simulink model "RunningLEDExample"  (R2015a)
settings: Solver=ode3  SolverMode=SingleTasking  StartTime=0.0  StopTime=inf  FixedStep=Ts  RelTol=1e-3
undefined symbols (not defined in the file): Ts
libraries: simulink x1
(part 2 of 2)

== system RunningLEDExample/Subsystem7/Subsystem3 ==
  In1 : Inport
  Constant4 : Constant  Value=15  OutDataTypeStr=uint8
  Constant5 : Constant  Value=0  OutDataTypeStr=uint8
  If : If  IfExpression=u1 == 81
  If Action Subsystem : Subsystem  TreatAsAtomicUnit=on
  If Action Subsystem1 : Subsystem  TreatAsAtomicUnit=on
  Merge : Merge
  Out1 : Outport  OutDataTypeStr=uint8
  wires:
  If/1 -> If Action Subsystem/Action
  If/2 -> If Action Subsystem1/Action
  In1/1 -> If/1
  Constant5/1 -> If Action Subsystem1/1(In1)
  Merge/1 -> Out1/1
  Constant4/1 -> If Action Subsystem/1(In1)
  If Action Subsystem/1(Out1) -> Merge/1
  If Action Subsystem1/1(Out1) -> Merge/2

== system RunningLEDExample/Subsystem7/Subsystem4 ==
  In1 : Inport
  Constant4 : Constant  Value=15  OutDataTypeStr=uint8
  Constant5 : Constant  Value=0  OutDataTypeStr=uint8
  If : If  IfExpression=u1 == 82
  If Action Subsystem : Subsystem  TreatAsAtomicUnit=on
  If Action Subsystem1 : Subsystem  TreatAsAtomicUnit=on
  Merge : Merge
  Out1 : Outport  OutDataTypeStr=uint8
  wires:
  If/1 -> If Action Subsystem/Action
  If/2 -> If Action Subsystem1/Action
  In1/1 -> If/1
  Constant5/1 -> If Action Subsystem1/1(In1)
  Merge/1 -> Out1/1
  Constant4/1 -> If Action Subsystem/1(In1)
  If Action Subsystem/1(Out1) -> Merge/1
  If Action Subsystem1/1(Out1) -> Merge/2

== system RunningLEDExample/Subsystem8/Subsystem ==
  In1 : Inport
  Constant4 : Constant  Value=15  OutDataTypeStr=uint8
  Constant5 : Constant  Value=0  OutDataTypeStr=uint8
  If : If  IfExpression=u1 == 96
  If Action Subsystem : Subsystem  TreatAsAtomicUnit=on
  If Action Subsystem1 : Subsystem  TreatAsAtomicUnit=on
  Merge : Merge
  Out1 : Outport  OutDataTypeStr=uint8
  wires:
  If/1 -> If Action Subsystem/Action
  If/2 -> If Action Subsystem1/Action
  In1/1 -> If/1
  Constant5/1 -> If Action Subsystem1/1(In1)
  Merge/1 -> Out1/1
  Constant4/1 -> If Action Subsystem/1(In1)
  If Action Subsystem/1(Out1) -> Merge/1
  If Action Subsystem1/1(Out1) -> Merge/2

== system RunningLEDExample/Subsystem8/Subsystem3 ==
  In1 : Inport
  Constant4 : Constant  Value=15  OutDataTypeStr=uint8
  Constant5 : Constant  Value=0  OutDataTypeStr=uint8
  If : If  IfExpression=u1 == 97
  If Action Subsystem : Subsystem  TreatAsAtomicUnit=on
  If Action Subsystem1 : Subsystem  TreatAsAtomicUnit=on
  Merge : Merge
  Out1 : Outport  OutDataTypeStr=uint8
  wires:
  If/1 -> If Action Subsystem/Action
  If/2 -> If Action Subsystem1/Action
  In1/1 -> If/1
  Constant5/1 -> If Action Subsystem1/1(In1)
  Merge/1 -> Out1/1
  Constant4/1 -> If Action Subsystem/1(In1)
  If Action Subsystem/1(Out1) -> Merge/1
  If Action Subsystem1/1(Out1) -> Merge/2

== system RunningLEDExample/Subsystem8/Subsystem4 ==
  In1 : Inport
  Constant4 : Constant  Value=15  OutDataTypeStr=uint8
  Constant5 : Constant  Value=0  OutDataTypeStr=uint8
  If : If  IfExpression=u1 == 98
  If Action Subsystem : Subsystem  TreatAsAtomicUnit=on
  If Action Subsystem1 : Subsystem  TreatAsAtomicUnit=on
  Merge : Merge
  Out1 : Outport  OutDataTypeStr=uint8
  wires:
  If/1 -> If Action Subsystem/Action
  If/2 -> If Action Subsystem1/Action
  In1/1 -> If/1
  Constant5/1 -> If Action Subsystem1/1(In1)
  Merge/1 -> Out1/1
  Constant4/1 -> If Action Subsystem/1(In1)
  If Action Subsystem/1(Out1) -> Merge/1
  If Action Subsystem1/1(Out1) -> Merge/2

== system RunningLEDExample/Subsystem9/Subsystem ==
  In1 : Inport
  Constant4 : Constant  Value=15  OutDataTypeStr=uint8
  Constant5 : Constant  Value=0  OutDataTypeStr=uint8
  If : If  IfExpression=u1 == 112
  If Action Subsystem : Subsystem  TreatAsAtomicUnit=on
  If Action Subsystem1 : Subsystem  TreatAsAtomicUnit=on
  Merge : Merge
  Out1 : Outport  OutDataTypeStr=uint8
  wires:
  If/1 -> If Action Subsystem/Action
  If/2 -> If Action Subsystem1/Action
  In1/1 -> If/1
  Constant5/1 -> If Action Subsystem1/1(In1)
  Merge/1 -> Out1/1
  Constant4/1 -> If Action Subsystem/1(In1)
  If Action Subsystem/1(Out1) -> Merge/1
  If Action Subsystem1/1(Out1) -> Merge/2

== system RunningLEDExample/Subsystem9/Subsystem3 ==
  In1 : Inport
  Constant4 : Constant  Value=15  OutDataTypeStr=uint8
  Constant5 : Constant  Value=0  OutDataTypeStr=uint8
  If : If  IfExpression=u1 == 113
  If Action Subsystem : Subsystem  TreatAsAtomicUnit=on
  If Action Subsystem1 : Subsystem  TreatAsAtomicUnit=on
  Merge : Merge
  Out1 : Outport  OutDataTypeStr=uint8
  wires:
  If/1 -> If Action Subsystem/Action
  If/2 -> If Action Subsystem1/Action
  In1/1 -> If/1
  Constant5/1 -> If Action Subsystem1/1(In1)
  Merge/1 -> Out1/1
  Constant4/1 -> If Action Subsystem/1(In1)
  If Action Subsystem/1(Out1) -> Merge/1
  If Action Subsystem1/1(Out1) -> Merge/2

== system RunningLEDExample/Subsystem9/Subsystem4 ==
  In1 : Inport
  Constant4 : Constant  Value=15  OutDataTypeStr=uint8
  Constant5 : Constant  Value=0  OutDataTypeStr=uint8
  If : If  IfExpression=u1 == 114
  If Action Subsystem : Subsystem  TreatAsAtomicUnit=on
  If Action Subsystem1 : Subsystem  TreatAsAtomicUnit=on
  Merge : Merge
  Out1 : Outport  OutDataTypeStr=uint8
  wires:
  If/1 -> If Action Subsystem/Action
  If/2 -> If Action Subsystem1/Action
  In1/1 -> If/1
  Constant5/1 -> If Action Subsystem1/1(In1)
  Merge/1 -> Out1/1
  Constant4/1 -> If Action Subsystem/1(In1)
  If Action Subsystem/1(Out1) -> Merge/1
  If Action Subsystem1/1(Out1) -> Merge/2

== system RunningLEDExample/Subsystem1/Subsystem/If Action Subsystem ==
  In1 : Inport
  Action Port : ActionPort  ActionType=then
  Out1 : Outport  OutDataTypeStr=uint8
  wires:
  In1/1 -> Out1/1

== system RunningLEDExample/Subsystem1/Subsystem/If Action Subsystem1 ==
  In1 : Inport
  Action Port : ActionPort  ActionType=else
  Out1 : Outport  OutDataTypeStr=uint8
  wires:
  In1/1 -> Out1/1

== system RunningLEDExample/Subsystem1/Subsystem3/If Action Subsystem ==
  In1 : Inport
  Action Port : ActionPort  ActionType=then
  Out1 : Outport  OutDataTypeStr=uint8
  wires:
  In1/1 -> Out1/1

== system RunningLEDExample/Subsystem1/Subsystem3/If Action Subsystem1 ==
  In1 : Inport
  Action Port : ActionPort  ActionType=else
  Out1 : Outport  OutDataTypeStr=uint8
  wires:
  In1/1 -> Out1/1

== system RunningLEDExample/Subsystem1/Subsystem4/If Action Subsystem ==
  In1 : Inport
  Action Port : ActionPort  ActionType=then
  Out1 : Outport  OutDataTypeStr=uint8
  wires:
  In1/1 -> Out1/1

== system RunningLEDExample/Subsystem1/Subsystem4/If Action Subsystem1 ==
  In1 : Inport
  Action Port : ActionPort  ActionType=else
  Out1 : Outport  OutDataTypeStr=uint8
  wires:
  In1/1 -> Out1/1

== system RunningLEDExample/Subsystem10/Subsystem/If Action Subsystem ==
  In1 : Inport
  Action Port : ActionPort  ActionType=then
  Out1 : Outport  OutDataTypeStr=uint8
  wires:
  In1/1 -> Out1/1

== system RunningLEDExample/Subsystem10/Subsystem/If Action Subsystem1 ==
  In1 : Inport
  Action Port : ActionPort  ActionType=else
  Out1 : Outport  OutDataTypeStr=uint8
  wires:
  In1/1 -> Out1/1

== system RunningLEDExample/Subsystem10/Subsystem3/If Action Subsystem ==
  In1 : Inport
  Action Port : ActionPort  ActionType=then
  Out1 : Outport  OutDataTypeStr=uint8
  wires:
  In1/1 -> Out1/1

== system RunningLEDExample/Subsystem10/Subsystem3/If Action Subsystem1 ==
  In1 : Inport
  Action Port : ActionPort  ActionType=else
  Out1 : Outport  OutDataTypeStr=uint8
  wires:
  In1/1 -> Out1/1

== system RunningLEDExample/Subsystem10/Subsystem4/If Action Subsystem ==
  In1 : Inport
  Action Port : ActionPort  ActionType=then
  Out1 : Outport  OutDataTypeStr=uint8
  wires:
  In1/1 -> Out1/1

== system RunningLEDExample/Subsystem10/Subsystem4/If Action Subsystem1 ==
  In1 : Inport
  Action Port : ActionPort  ActionType=else
  Out1 : Outport  OutDataTypeStr=uint8
  wires:
  In1/1 -> Out1/1

== system RunningLEDExample/Subsystem11/Subsystem/If Action Subsystem ==
  In1 : Inport
  Action Port : ActionPort  ActionType=then
  Out1 : Outport  OutDataTypeStr=uint8
  wires:
  In1/1 -> Out1/1

== system RunningLEDExample/Subsystem11/Subsystem/If Action Subsystem1 ==
  In1 : Inport
  Action Port : ActionPort  ActionType=else
  Out1 : Outport  OutDataTypeStr=uint8
  wires:
  In1/1 -> Out1/1

== system RunningLEDExample/Subsystem11/Subsystem3/If Action Subsystem ==
  In1 : Inport
  Action Port : ActionPort  ActionType=then
  Out1 : Outport  OutDataTypeStr=uint8
  wires:
  In1/1 -> Out1/1

== system RunningLEDExample/Subsystem11/Subsystem3/If Action Subsystem1 ==
  In1 : Inport
  Action Port : ActionPort  ActionType=else
  Out1 : Outport  OutDataTypeStr=uint8
  wires:
  In1/1 -> Out1/1

== system RunningLEDExample/Subsystem11/Subsystem4/If Action Subsystem ==
  In1 : Inport
  Action Port : ActionPort  ActionType=then
  Out1 : Outport  OutDataTypeStr=uint8
  wires:
  In1/1 -> Out1/1

== system RunningLEDExample/Subsystem11/Subsystem4/If Action Subsystem1 ==
  In1 : Inport
  Action Port : ActionPort  ActionType=else
  Out1 : Outport  OutDataTypeStr=uint8
  wires:
  In1/1 -> Out1/1

== system RunningLEDExample/Subsystem12/Subsystem/If Action Subsystem ==
  In1 : Inport
  Action Port : ActionPort  ActionType=then
  Out1 : Outport  OutDataTypeStr=uint8
  wires:
  In1/1 -> Out1/1

== system RunningLEDExample/Subsystem12/Subsystem/If Action Subsystem1 ==
  In1 : Inport
  Action Port : ActionPort  ActionType=else
  Out1 : Outport  OutDataTypeStr=uint8
  wires:
  In1/1 -> Out1/1

== system RunningLEDExample/Subsystem12/Subsystem3/If Action Subsystem ==
  In1 : Inport
  Action Port : ActionPort  ActionType=then
  Out1 : Outport  OutDataTypeStr=uint8
  wires:
  In1/1 -> Out1/1

== system RunningLEDExample/Subsystem12/Subsystem3/If Action Subsystem1 ==
  In1 : Inport
  Action Port : ActionPort  ActionType=else
  Out1 : Outport  OutDataTypeStr=uint8
  wires:
  In1/1 -> Out1/1

== system RunningLEDExample/Subsystem12/Subsystem4/If Action Subsystem ==
  In1 : Inport
  Action Port : ActionPort  ActionType=then
  Out1 : Outport  OutDataTypeStr=uint8
  wires:
  In1/1 -> Out1/1

== system RunningLEDExample/Subsystem12/Subsystem4/If Action Subsystem1 ==
  In1 : Inport
  Action Port : ActionPort  ActionType=else
  Out1 : Outport  OutDataTypeStr=uint8
  wires:
  In1/1 -> Out1/1

== system RunningLEDExample/Subsystem13/Subsystem/If Action Subsystem ==
  In1 : Inport
  Action Port : ActionPort  ActionType=then
  Out1 : Outport  OutDataTypeStr=uint8
  wires:
  In1/1 -> Out1/1

== system RunningLEDExample/Subsystem13/Subsystem/If Action Subsystem1 ==
  In1 : Inport
  Action Port : ActionPort  ActionType=else
  Out1 : Outport  OutDataTypeStr=uint8
  wires:
  In1/1 -> Out1/1

== system RunningLEDExample/Subsystem13/Subsystem3/If Action Subsystem ==
  In1 : Inport
  Action Port : ActionPort  ActionType=then
  Out1 : Outport  OutDataTypeStr=uint8
  wires:
  In1/1 -> Out1/1

== system RunningLEDExample/Subsystem13/Subsystem3/If Action Subsystem1 ==
  In1 : Inport
  Action Port : ActionPort  ActionType=else
  Out1 : Outport  OutDataTypeStr=uint8
  wires:
  In1/1 -> Out1/1

== system RunningLEDExample/Subsystem13/Subsystem4/If Action Subsystem ==
  In1 : Inport
  Action Port : ActionPort  ActionType=then
  Out1 : Outport  OutDataTypeStr=uint8
  wires:
  In1/1 -> Out1/1

== system RunningLEDExample/Subsystem13/Subsystem4/If Action Subsystem1 ==
  In1 : Inport
  Action Port : ActionPort  ActionType=else
  Out1 : Outport  OutDataTypeStr=uint8
  wires:
  In1/1 -> Out1/1

== system RunningLEDExample/Subsystem14/Subsystem/If Action Subsystem ==
  In1 : Inport
  Action Port : ActionPort  ActionType=then
  Out1 : Outport  OutDataTypeStr=uint8
  wires:
  In1/1 -> Out1/1

== system RunningLEDExample/Subsystem14/Subsystem/If Action Subsystem1 ==
  In1 : Inport
  Action Port : ActionPort  ActionType=else
  Out1 : Outport  OutDataTypeStr=uint8
  wires:
  In1/1 -> Out1/1

== system RunningLEDExample/Subsystem14/Subsystem3/If Action Subsystem ==
  In1 : Inport
  Action Port : ActionPort  ActionType=then
  Out1 : Outport  OutDataTypeStr=uint8
  wires:
  In1/1 -> Out1/1

== system RunningLEDExample/Subsystem14/Subsystem3/If Action Subsystem1 ==
  In1 : Inport
  Action Port : ActionPort  ActionType=else
  Out1 : Outport  OutDataTypeStr=uint8
  wires:
  In1/1 -> Out1/1

== system RunningLEDExample/Subsystem14/Subsystem4/If Action Subsystem ==
  In1 : Inport
  Action Port : ActionPort  ActionType=then
  Out1 : Outport  OutDataTypeStr=uint8
  wires:
  In1/1 -> Out1/1

== system RunningLEDExample/Subsystem14/Subsystem4/If Action Subsystem1 ==
  In1 : Inport
  Action Port : ActionPort  ActionType=else
  Out1 : Outport  OutDataTypeStr=uint8
  wires:
  In1/1 -> Out1/1

== system RunningLEDExample/Subsystem15/Subsystem/If Action Subsystem ==
  In1 : Inport
  Action Port : ActionPort  ActionType=then
  Out1 : Outport  OutDataTypeStr=uint8
  wires:
  In1/1 -> Out1/1

== system RunningLEDExample/Subsystem15/Subsystem/If Action Subsystem1 ==
  In1 : Inport
  Action Port : ActionPort  ActionType=else
  Out1 : Outport  OutDataTypeStr=uint8
  wires:
  In1/1 -> Out1/1

== system RunningLEDExample/Subsystem15/Subsystem3/If Action Subsystem ==
  In1 : Inport
  Action Port : ActionPort  ActionType=then
  Out1 : Outport  OutDataTypeStr=uint8
  wires:
  In1/1 -> Out1/1

== system RunningLEDExample/Subsystem15/Subsystem3/If Action Subsystem1 ==
  In1 : Inport
  Action Port : ActionPort  ActionType=else
  Out1 : Outport  OutDataTypeStr=uint8
  wires:
  In1/1 -> Out1/1

== system RunningLEDExample/Subsystem15/Subsystem4/If Action Subsystem ==
  In1 : Inport
  Action Port : ActionPort  ActionType=then
  Out1 : Outport  OutDataTypeStr=uint8
  wires:
  In1/1 -> Out1/1

== system RunningLEDExample/Subsystem15/Subsystem4/If Action Subsystem1 ==
  In1 : Inport
  Action Port : ActionPort  ActionType=else
  Out1 : Outport  OutDataTypeStr=uint8
  wires:
  In1/1 -> Out1/1

== system RunningLEDExample/Subsystem16/Subsystem/If Action Subsystem ==
  In1 : Inport
  Action Port : ActionPort  ActionType=then
  Out1 : Outport  OutDataTypeStr=uint8
  wires:
  In1/1 -> Out1/1

== system RunningLEDExample/Subsystem16/Subsystem/If Action Subsystem1 ==
  In1 : Inport
  Action Port : ActionPort  ActionType=else
  Out1 : Outport  OutDataTypeStr=uint8
  wires:
  In1/1 -> Out1/1

== system RunningLEDExample/Subsystem16/Subsystem3/If Action Subsystem ==
  In1 : Inport
  Action Port : ActionPort  ActionType=then
  Out1 : Outport  OutDataTypeStr=uint8
  wires:
  In1/1 -> Out1/1

== system RunningLEDExample/Subsystem16/Subsystem3/If Action Subsystem1 ==
  In1 : Inport
  Action Port : ActionPort  ActionType=else
  Out1 : Outport  OutDataTypeStr=uint8
  wires:
  In1/1 -> Out1/1

== system RunningLEDExample/Subsystem16/Subsystem4/If Action Subsystem ==
  In1 : Inport
  Action Port : ActionPort  ActionType=then
  Out1 : Outport  OutDataTypeStr=uint8
  wires:
  In1/1 -> Out1/1

== system RunningLEDExample/Subsystem16/Subsystem4/If Action Subsystem1 ==
  In1 : Inport
  Action Port : ActionPort  ActionType=else
  Out1 : Outport  OutDataTypeStr=uint8
  wires:
  In1/1 -> Out1/1

== system RunningLEDExample/Subsystem17/Subsystem/If Action Subsystem ==
  In1 : Inport
  Action Port : ActionPort  ActionType=then
  Out1 : Outport  OutDataTypeStr=uint8
  wires:
  In1/1 -> Out1/1

== system RunningLEDExample/Subsystem17/Subsystem/If Action Subsystem1 ==
  In1 : Inport
  Action Port : ActionPort  ActionType=else
  Out1 : Outport  OutDataTypeStr=uint8
  wires:
  In1/1 -> Out1/1

== system RunningLEDExample/Subsystem17/Subsystem3/If Action Subsystem ==
  In1 : Inport
  Action Port : ActionPort  ActionType=then
  Out1 : Outport  OutDataTypeStr=uint8
  wires:
  In1/1 -> Out1/1

== system RunningLEDExample/Subsystem17/Subsystem3/If Action Subsystem1 ==
  In1 : Inport
  Action Port : ActionPort  ActionType=else
  Out1 : Outport  OutDataTypeStr=uint8
  wires:
  In1/1 -> Out1/1

== system RunningLEDExample/Subsystem17/Subsystem4/If Action Subsystem ==
  In1 : Inport
  Action Port : ActionPort  ActionType=then
  Out1 : Outport  OutDataTypeStr=uint8
  wires:
  In1/1 -> Out1/1

== system RunningLEDExample/Subsystem17/Subsystem4/If Action Subsystem1 ==
  In1 : Inport
  Action Port : ActionPort  ActionType=else
  Out1 : Outport  OutDataTypeStr=uint8
  wires:
  In1/1 -> Out1/1

== system RunningLEDExample/Subsystem3/Subsystem/If Action Subsystem ==
  In1 : Inport
  Action Port : ActionPort  ActionType=then
  Out1 : Outport  OutDataTypeStr=uint8
  wires:
  In1/1 -> Out1/1

== system RunningLEDExample/Subsystem3/Subsystem/If Action Subsystem1 ==
  In1 : Inport
  Action Port : ActionPort  ActionType=else
  Out1 : Outport  OutDataTypeStr=uint8
  wires:
  In1/1 -> Out1/1

== system RunningLEDExample/Subsystem3/Subsystem3/If Action Subsystem ==
  In1 : Inport
  Action Port : ActionPort  ActionType=then
  Out1 : Outport  OutDataTypeStr=uint8
  wires:
  In1/1 -> Out1/1

== system RunningLEDExample/Subsystem3/Subsystem3/If Action Subsystem1 ==
  In1 : Inport
  Action Port : ActionPort  ActionType=else
  Out1 : Outport  OutDataTypeStr=uint8
  wires:
  In1/1 -> Out1/1

== system RunningLEDExample/Subsystem3/Subsystem4/If Action Subsystem ==
  In1 : Inport
  Action Port : ActionPort  ActionType=then
  Out1 : Outport  OutDataTypeStr=uint8
  wires:
  In1/1 -> Out1/1

== system RunningLEDExample/Subsystem3/Subsystem4/If Action Subsystem1 ==
  In1 : Inport
  Action Port : ActionPort  ActionType=else
  Out1 : Outport  OutDataTypeStr=uint8
  wires:
  In1/1 -> Out1/1

== system RunningLEDExample/Subsystem4/Subsystem/If Action Subsystem ==
  In1 : Inport
  Action Port : ActionPort  ActionType=then
  Out1 : Outport  OutDataTypeStr=uint8
  wires:
  In1/1 -> Out1/1

== system RunningLEDExample/Subsystem4/Subsystem/If Action Subsystem1 ==
  In1 : Inport
  Action Port : ActionPort  ActionType=else
  Out1 : Outport  OutDataTypeStr=uint8
  wires:
  In1/1 -> Out1/1

== system RunningLEDExample/Subsystem4/Subsystem3/If Action Subsystem ==
  In1 : Inport
  Action Port : ActionPort  ActionType=then
  Out1 : Outport  OutDataTypeStr=uint8
  wires:
  In1/1 -> Out1/1

== system RunningLEDExample/Subsystem4/Subsystem3/If Action Subsystem1 ==
  In1 : Inport
  Action Port : ActionPort  ActionType=else
  Out1 : Outport  OutDataTypeStr=uint8
  wires:
  In1/1 -> Out1/1

== system RunningLEDExample/Subsystem4/Subsystem4/If Action Subsystem ==
  In1 : Inport
  Action Port : ActionPort  ActionType=then
  Out1 : Outport  OutDataTypeStr=uint8
  wires:
  In1/1 -> Out1/1

== system RunningLEDExample/Subsystem4/Subsystem4/If Action Subsystem1 ==
  In1 : Inport
  Action Port : ActionPort  ActionType=else
  Out1 : Outport  OutDataTypeStr=uint8
  wires:
  In1/1 -> Out1/1

== system RunningLEDExample/Subsystem5/Subsystem/If Action Subsystem ==
  In1 : Inport
  Action Port : ActionPort  ActionType=then
  Out1 : Outport  OutDataTypeStr=uint8
  wires:
  In1/1 -> Out1/1

== system RunningLEDExample/Subsystem5/Subsystem/If Action Subsystem1 ==
  In1 : Inport
  Action Port : ActionPort  ActionType=else
  Out1 : Outport  OutDataTypeStr=uint8
  wires:
  In1/1 -> Out1/1

== system RunningLEDExample/Subsystem5/Subsystem3/If Action Subsystem ==
  In1 : Inport
  Action Port : ActionPort  ActionType=then
  Out1 : Outport  OutDataTypeStr=uint8
  wires:
  In1/1 -> Out1/1

== system RunningLEDExample/Subsystem5/Subsystem3/If Action Subsystem1 ==
  In1 : Inport
  Action Port : ActionPort  ActionType=else
  Out1 : Outport  OutDataTypeStr=uint8
  wires:
  In1/1 -> Out1/1

== system RunningLEDExample/Subsystem5/Subsystem4/If Action Subsystem ==
  In1 : Inport
  Action Port : ActionPort  ActionType=then
  Out1 : Outport  OutDataTypeStr=uint8
  wires:
  In1/1 -> Out1/1

== system RunningLEDExample/Subsystem5/Subsystem4/If Action Subsystem1 ==
  In1 : Inport
  Action Port : ActionPort  ActionType=else
  Out1 : Outport  OutDataTypeStr=uint8
  wires:
  In1/1 -> Out1/1

== system RunningLEDExample/Subsystem6/Subsystem/If Action Subsystem ==
  In1 : Inport
  Action Port : ActionPort  ActionType=then
  Out1 : Outport  OutDataTypeStr=uint8
  wires:
  In1/1 -> Out1/1

== system RunningLEDExample/Subsystem6/Subsystem/If Action Subsystem1 ==
  In1 : Inport
  Action Port : ActionPort  ActionType=else
  Out1 : Outport  OutDataTypeStr=uint8
  wires:
  In1/1 -> Out1/1

== system RunningLEDExample/Subsystem6/Subsystem3/If Action Subsystem ==
  In1 : Inport
  Action Port : ActionPort  ActionType=then
  Out1 : Outport  OutDataTypeStr=uint8
  wires:
  In1/1 -> Out1/1

== system RunningLEDExample/Subsystem6/Subsystem3/If Action Subsystem1 ==
  In1 : Inport
  Action Port : ActionPort  ActionType=else
  Out1 : Outport  OutDataTypeStr=uint8
  wires:
  In1/1 -> Out1/1

== system RunningLEDExample/Subsystem6/Subsystem4/If Action Subsystem ==
  In1 : Inport
  Action Port : ActionPort  ActionType=then
  Out1 : Outport  OutDataTypeStr=uint8
  wires:
  In1/1 -> Out1/1

== system RunningLEDExample/Subsystem6/Subsystem4/If Action Subsystem1 ==
  In1 : Inport
  Action Port : ActionPort  ActionType=else
  Out1 : Outport  OutDataTypeStr=uint8
  wires:
  In1/1 -> Out1/1

== system RunningLEDExample/Subsystem7/Subsystem/If Action Subsystem ==
  In1 : Inport
  Action Port : ActionPort  ActionType=then
  Out1 : Outport  OutDataTypeStr=uint8
  wires:
  In1/1 -> Out1/1

== system RunningLEDExample/Subsystem7/Subsystem/If Action Subsystem1 ==
  In1 : Inport
  Action Port : ActionPort  ActionType=else
  Out1 : Outport  OutDataTypeStr=uint8
  wires:
  In1/1 -> Out1/1

== system RunningLEDExample/Subsystem7/Subsystem3/If Action Subsystem ==
  In1 : Inport
  Action Port : ActionPort  ActionType=then
  Out1 : Outport  OutDataTypeStr=uint8
  wires:
  In1/1 -> Out1/1

== system RunningLEDExample/Subsystem7/Subsystem3/If Action Subsystem1 ==
  In1 : Inport
  Action Port : ActionPort  ActionType=else
  Out1 : Outport  OutDataTypeStr=uint8
  wires:
  In1/1 -> Out1/1

== system RunningLEDExample/Subsystem7/Subsystem4/If Action Subsystem ==
  In1 : Inport
  Action Port : ActionPort  ActionType=then
  Out1 : Outport  OutDataTypeStr=uint8
  wires:
  In1/1 -> Out1/1

== system RunningLEDExample/Subsystem7/Subsystem4/If Action Subsystem1 ==
  In1 : Inport
  Action Port : ActionPort  ActionType=else
  Out1 : Outport  OutDataTypeStr=uint8
  wires:
  In1/1 -> Out1/1

== system RunningLEDExample/Subsystem8/Subsystem/If Action Subsystem ==
  In1 : Inport
  Action Port : ActionPort  ActionType=then
  Out1 : Outport  OutDataTypeStr=uint8
  wires:
  In1/1 -> Out1/1

== system RunningLEDExample/Subsystem8/Subsystem/If Action Subsystem1 ==
  In1 : Inport
  Action Port : ActionPort  ActionType=else
  Out1 : Outport  OutDataTypeStr=uint8
  wires:
  In1/1 -> Out1/1

== system RunningLEDExample/Subsystem8/Subsystem3/If Action Subsystem ==
  In1 : Inport
  Action Port : ActionPort  ActionType=then
  Out1 : Outport  OutDataTypeStr=uint8
  wires:
  In1/1 -> Out1/1

== system RunningLEDExample/Subsystem8/Subsystem3/If Action Subsystem1 ==
  In1 : Inport
  Action Port : ActionPort  ActionType=else
  Out1 : Outport  OutDataTypeStr=uint8
  wires:
  In1/1 -> Out1/1

== system RunningLEDExample/Subsystem8/Subsystem4/If Action Subsystem ==
  In1 : Inport
  Action Port : ActionPort  ActionType=then
  Out1 : Outport  OutDataTypeStr=uint8
  wires:
  In1/1 -> Out1/1

== system RunningLEDExample/Subsystem8/Subsystem4/If Action Subsystem1 ==
  In1 : Inport
  Action Port : ActionPort  ActionType=else
  Out1 : Outport  OutDataTypeStr=uint8
  wires:
  In1/1 -> Out1/1

== system RunningLEDExample/Subsystem9/Subsystem/If Action Subsystem ==
  In1 : Inport
  Action Port : ActionPort  ActionType=then
  Out1 : Outport  OutDataTypeStr=uint8
  wires:
  In1/1 -> Out1/1

== system RunningLEDExample/Subsystem9/Subsystem/If Action Subsystem1 ==
  In1 : Inport
  Action Port : ActionPort  ActionType=else
  Out1 : Outport  OutDataTypeStr=uint8
  wires:
  In1/1 -> Out1/1

== system RunningLEDExample/Subsystem9/Subsystem3/If Action Subsystem ==
  In1 : Inport
  Action Port : ActionPort  ActionType=then
  Out1 : Outport  OutDataTypeStr=uint8
  wires:
  In1/1 -> Out1/1

== system RunningLEDExample/Subsystem9/Subsystem3/If Action Subsystem1 ==
  In1 : Inport
  Action Port : ActionPort  ActionType=else
  Out1 : Outport  OutDataTypeStr=uint8
  wires:
  In1/1 -> Out1/1

== system RunningLEDExample/Subsystem9/Subsystem4/If Action Subsystem ==
  In1 : Inport
  Action Port : ActionPort  ActionType=then
  Out1 : Outport  OutDataTypeStr=uint8
  wires:
  In1/1 -> Out1/1

== system RunningLEDExample/Subsystem9/Subsystem4/If Action Subsystem1 ==
  In1 : Inport
  Action Port : ActionPort  ActionType=else
  Out1 : Outport  OutDataTypeStr=uint8
  wires:
  In1/1 -> Out1/1

== matlab function RunningLEDExample/Set RGB LED2 ==
  data: led_index parameter uint8 [0..15]; r input uint8 [0..15]; g input uint8 [0..15]; b input uint8 [0..15]
function rgb_led(led_index, r, g, b)

if strcmp(coder.target, 'rtw')
    coder.ceval('rgb_leds_wrapper', led_index, r, g, b);
end

== matlab function RunningLEDExample/Set RGB LED3 ==
  data: led_index parameter uint8 [0..15]; r input uint8 [0..15]; g input uint8 [0..15]; b input uint8 [0..15]
function rgb_led(led_index, r, g, b)

if strcmp(coder.target, 'rtw')
    coder.ceval('rgb_leds_wrapper', led_index, r, g, b);
end

== matlab function RunningLEDExample/Set RGB LED ==
  data: led_index parameter uint8 [0..15]; r input uint8 [0..15]; g input uint8 [0..15]; b input uint8 [0..15]
function rgb_led(led_index, r, g, b)

if strcmp(coder.target, 'rtw')
    coder.ceval('rgb_leds_wrapper', led_index, r, g, b);
end

== matlab function RunningLEDExample/Set RGB LED1 ==
  data: led_index parameter uint8 [0..15]; r input uint8 [0..15]; g input uint8 [0..15]; b input uint8 [0..15]
function rgb_led(led_index, r, g, b)

if strcmp(coder.target, 'rtw')
    coder.ceval('rgb_leds_wrapper', led_index, r, g, b);
end

== matlab function RunningLEDExample/Set RGB LED4 ==
  data: led_index parameter uint8 [0..15]; r input uint8 [0..15]; g input uint8 [0..15]; b input uint8 [0..15]
function rgb_led(led_index, r, g, b)

if strcmp(coder.target, 'rtw')
    coder.ceval('rgb_leds_wrapper', led_index, r, g, b);
end

== matlab function RunningLEDExample/Set RGB LED5 ==
  data: led_index parameter uint8 [0..15]; r input uint8 [0..15]; g input uint8 [0..15]; b input uint8 [0..15]
function rgb_led(led_index, r, g, b)

if strcmp(coder.target, 'rtw')
    coder.ceval('rgb_leds_wrapper', led_index, r, g, b);
end

== matlab function RunningLEDExample/Set RGB LED6 ==
  data: led_index parameter uint8 [0..15]; r input uint8 [0..15]; g input uint8 [0..15]; b input uint8 [0..15]
function rgb_led(led_index, r, g, b)

if strcmp(coder.target, 'rtw')
    coder.ceval('rgb_leds_wrapper', led_index, r, g, b);
end

== matlab function RunningLEDExample/Set RGB LED7 ==
  data: led_index parameter uint8 [0..15]; r input uint8 [0..15]; g input uint8 [0..15]; b input uint8 [0..15]
function rgb_led(led_index, r, g, b)

if strcmp(coder.target, 'rtw')
    coder.ceval('rgb_leds_wrapper', led_index, r, g, b);
end

== matlab function RunningLEDExample/Set RGB LED8 ==
  data: led_index parameter uint8 [0..15]; r input uint8 [0..15]; g input uint8 [0..15]; b input uint8 [0..15]
function rgb_led(led_index, r, g, b)

if strcmp(coder.target, 'rtw')
    coder.ceval('rgb_leds_wrapper', led_index, r, g, b);
end

== matlab function RunningLEDExample/Set RGB LED10 ==
  data: led_index parameter uint8 [0..15]; r input uint8 [0..15]; g input uint8 [0..15]; b input uint8 [0..15]
function rgb_led(led_index, r, g, b)

if strcmp(coder.target, 'rtw')
    coder.ceval('rgb_leds_wrapper', led_index, r, g, b);
end

== matlab function RunningLEDExample/Set RGB LED11 ==
  data: led_index parameter uint8 [0..15]; r input uint8 [0..15]; g input uint8 [0..15]; b input uint8 [0..15]
function rgb_led(led_index, r, g, b)

if strcmp(coder.target, 'rtw')
    coder.ceval('rgb_leds_wrapper', led_index, r, g, b);
end

== matlab function RunningLEDExample/Set RGB LED9 ==
  data: led_index parameter uint8 [0..15]; r input uint8 [0..15]; g input uint8 [0..15]; b input uint8 [0..15]
function rgb_led(led_index, r, g, b)

if strcmp(coder.target, 'rtw')
    coder.ceval('rgb_leds_wrapper', led_index, r, g, b);
end

== matlab function RunningLEDExample/Set RGB LED12 ==
  data: led_index parameter uint8 [0..15]; r input uint8 [0..15]; g input uint8 [0..15]; b input uint8 [0..15]
function rgb_led(led_index, r, g, b)

if strcmp(coder.target, 'rtw')
    coder.ceval('rgb_leds_wrapper', led_index, r, g, b);
end

== matlab function RunningLEDExample/Set RGB LED13 ==
  data: led_index parameter uint8 [0..15]; r input uint8 [0..15]; g input uint8 [0..15]; b input uint8 [0..15]
function rgb_led(led_index, r, g, b)

if strcmp(coder.target, 'rtw')
    coder.ceval('rgb_leds_wrapper', led_index, r, g, b);
end

== matlab function RunningLEDExample/Set RGB LED14 ==
  data: led_index parameter uint8 [0..15]; r input uint8 [0..15]; g input uint8 [0..15]; b input uint8 [0..15]
function rgb_led(led_index, r, g, b)

if strcmp(coder.target, 'rtw')
    coder.ceval('rgb_leds_wrapper', led_index, r, g, b);
end

== matlab function RunningLEDExample/Set RGB LED15 ==
  data: led_index parameter uint8 [0..15]; r input uint8 [0..15]; g input uint8 [0..15]; b input uint8 [0..15]
function rgb_led(led_index, r, g, b)

if strcmp(coder.target, 'rtw')
    coder.ceval('rgb_leds_wrapper', led_index, r, g, b);
end
